simulink model "ROS2Simulink"  (R2023b)
settings: Solver=FixedStepAuto  StartTime=0.0  StopTime=inf  RelTol=1e-3
undefined symbols (not defined in the file): Angular, Linear, Velocity
libraries: robotlib x7
settings Model: Creator=Renzhaofu  LastModifiedBy=Renzhaofu
settings OptimizationCC: EnhancedBackFolding=on  PassReuseOutputArgsAs=Individual arguments  ZeroExternalMemoryAtStartup=off  ZeroInternalMemoryAtStartup=off  MaxStackSize=64  OptimizeBlockOrder=speed  DifferentSizesBufferReuse=on  OptimizationCustomize=off  EfficientTunableParamExpr=on
settings DebuggingCC: ParameterTunabilityLossMsg=error
settings HardwareCC: ProdBitPerPointer=32  ProdBitPerSizeT=32  ProdBitPerPtrDiffT=32  ProdLargestAtomicFloat=None  ProdIntDivRoundTo=Undefined  ProdEndianess=Unspecified  ProdWordSize=32  ProdHWDeviceType=Generic->Unspecified (assume 32-bit Generic)
settings SFSimCC: MATLABDynamicMemAlloc=off
settings RTWCC: Description=Embedded Coder  SystemTargetFile=ert.tlc  HardwareBoard=Robot Operating System (ROS)  TLCOptions="-aInlineSetEventsForThisBaseRateFcn=TLC_FALSE -aSuppressMultiTaskScheduler=TLC_FALSE  -aRateBasedStepFcn=0"  TemplateMakefile=ert_default_tmf  Toolchain=Catkin  TargetLang=C++
settings CodeAppCC: ForceParamTrailComments=on  IgnoreCustomStorageClasses=off  OperatorAnnotations=on  SimulinkDataObjDesc=on  SFDataObjDesc=on  InsertBlockDesc=on

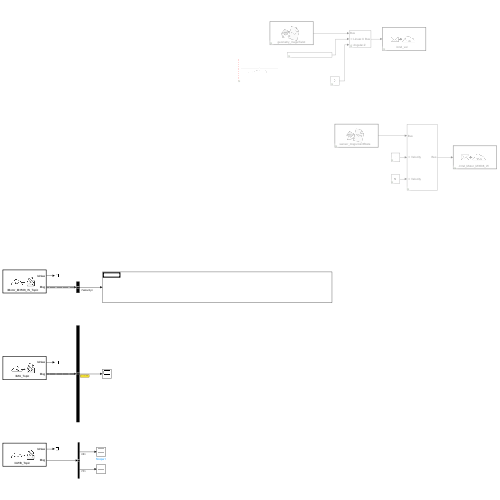
[thumbnail: Simulink's stored preview of the top-level diagram]
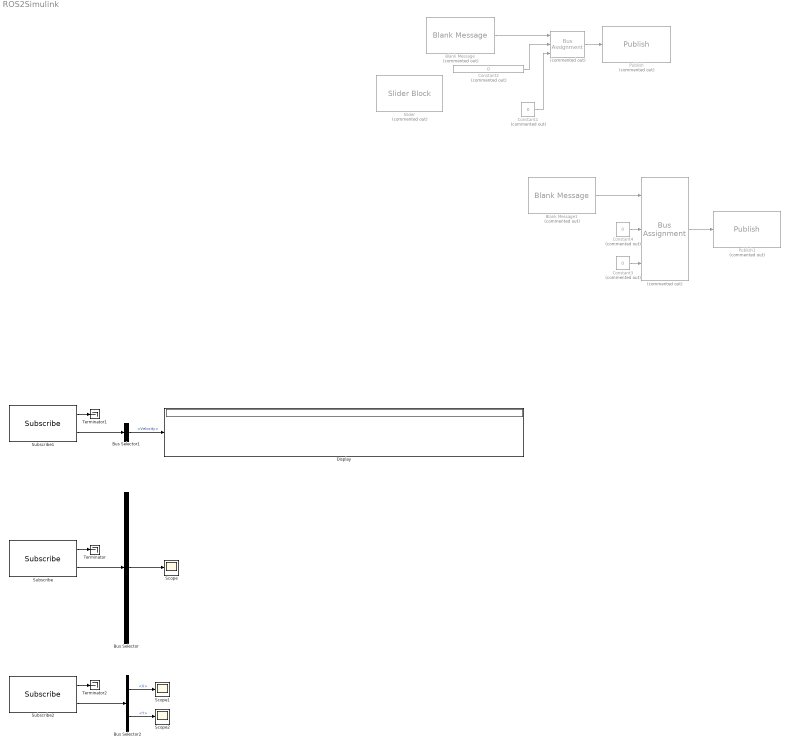
== system ROS2Simulink ==
  " " : BusAssignment  Commented=on  AssignedSignals=Linear.X,Angular.Z
  " " : BusAssignment  Commented=on  AssignedSignals=Velocity,Velocity
  Blank Message : robotlib/Blank Message  Commented=on  messageClass=Message  entityType=geometry_msgs/Twist  messageType=geometry_msgs/Twist  SampleTime=inf  legacyBusStruct=off
  Blank Message1 : robotlib/Blank Message  Commented=on  messageClass=Message  entityType=sensor_msgs/JointState  messageType=sensor_msgs/JointState  SampleTime=inf  legacyBusStruct=off
  Bus Selector : BusSelector  OutputSignals=Orientation.Z  OutputAsBus=on
  Bus Selector1 : BusSelector  OutputSignals=Velocity
  Bus Selector2 : BusSelector  OutputSignals=X,Y
  Constant{1..4} (4 alike) : Constant  Commented=on  Value=0
  Display : Display
  Publish : robotlib/Publish  Commented=on  topicSource=Select from ROS network  topic=/cmd_vel  messageType=geometry_msgs/Twist  legacyBusStruct=off  messageQueueLength=1
  Publish1 : robotlib/Publish  Commented=on  topicSource=Select from ROS network  topic=/cmd_Motor_M3508_W  messageType=sensor_msgs/JointState  legacyBusStruct=off  messageQueueLength=4
  Scope : Scope
  Scope1 : Scope
  Scope2 : Scope
  Slider : SliderBlock  Commented=on  LabelPosition=Hide  ScaleMin=-0.3  ScaleMax=+0.3
  Subscribe : robotlib/Subscribe  topicSource=Select from ROS network  topic=/IMU_Topic  messageType=sensor_msgs/Imu  SampleTime=0.1  legacyBusStruct=off  messageQueueLength=1
  Subscribe1 : robotlib/Subscribe  topicSource=Select from ROS network  topic=/Motor_M3508_W_Topic  messageType=sensor_msgs/JointState  SampleTime=0.1  legacyBusStruct=off  messageQueueLength=1
  Subscribe2 : robotlib/Subscribe  topicSource=Select from ROS network  topic=/UWB_Topic  messageType=geometry_msgs/Point  SampleTime=0.1  legacyBusStruct=off  messageQueueLength=1
  Terminator : Terminator
  Terminator1 : Terminator
  Terminator2 : Terminator
  wires:
  Blank Message/1 -> " "/1
  " "/1 -> Publish/1
  Constant1/1 -> " "/3
  Constant2/1 -> " "/2
  Blank Message1/1 -> " "/1
  " "/1 -> Publish1/1
  Constant3/1 -> " "/3
  Constant4/1 -> " "/2
  Subscribe/2 -> Bus Selector/1
  Subscribe/1 -> Terminator/1
  Bus Selector/1 -> Scope/1
  Subscribe1/1 -> Terminator1/1
  Subscribe1/2 -> Bus Selector1/1
  Bus Selector1/1 -> Display/1  "<Velocity>"
  Subscribe2/1 -> Terminator2/1
  Subscribe2/2 -> Bus Selector2/1
  Bus Selector2/1 -> Scope1/1  "<X>"
  Bus Selector2/2 -> Scope2/1  "<Y>"
